simulink model "nextpilot_simulation"  (R2024b)
settings: Solver=FixedStepAuto  StartTime=0.0  StopTime=10.0  FixedStep=5/1000  RelTol=1e-3
libraries: aerolibfltsims x1
settings Model: DataDictionary=nextpilot_datadict.sldd  Creator=zhanfuyu  LastModifiedBy=CETCA
settings SolverCC: MinimalZcImpactIntegration=on
settings OptimizationCC: ReuseModelBlockBuffer=off
settings DebuggingCC: ReadBeforeWriteMsg=DisableAll  WriteAfterWriteMsg=DisableAll  WriteAfterReadMsg=DisableAll  MultiTaskDSMMsg=none
settings ModelReferenceCC: UpdateModelReferenceTargets=IfOutOfDate  EnableParallelModelReferenceBuilds=on
settings SFSimCC: SFSimEcho=off
settings RTWCC: GPUComputeCapability=3.5

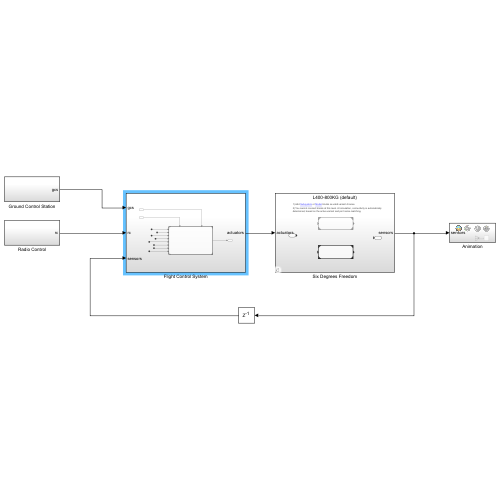
[thumbnail: Simulink's stored preview of the top-level diagram]
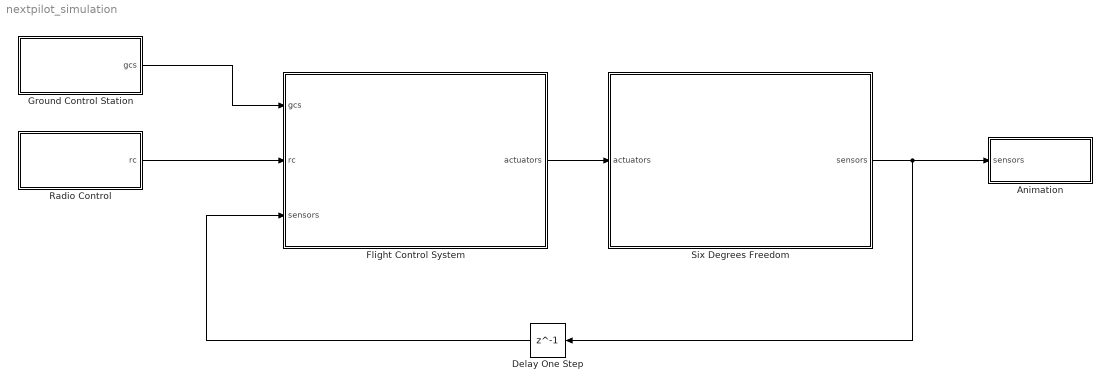
== system nextpilot_simulation ==
  Animation : Subsystem
  Delay One Step : Delay  DelayLength=1
  Flight Control System : Subsystem
  Ground Control Station : Subsystem
  Radio Control : Subsystem
  Six Degrees Freedom : Subsystem  Variant=on
  wires:
  Six Degrees Freedom/1(sensors) -> Delay One Step/1, Animation/1(sensors)
  Radio Control/1(rc) -> Flight Control System/2(rc)
  Ground Control Station/1(gcs) -> Flight Control System/1(gcs)
  Flight Control System/1(actuators) -> Six Degrees Freedom/1(actuators)
  Delay One Step/1 -> Flight Control System/3(sensors)

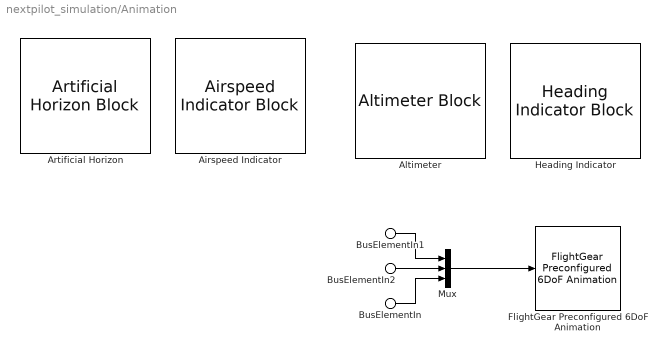
== system nextpilot_simulation/Animation ==
  BusElementIn : Inport  PortName=sensors  Element=states.aircraft.attitude.phi_theta_psi
  BusElementIn1 : Inport  PortName=sensors  Element=states.aircraft.position.lat_lon
  BusElementIn2 : Inport  PortName=sensors  Element=states.aircraft.position.alt
  Airspeed Indicator : AirspeedIndicatorBlock
  Altimeter : AltimeterBlock
  Artificial Horizon : ArtificialHorizonBlock  LabelPosition=Hide
  FlightGear Preconfigured 6DoF Animation : aerolibfltsims/FlightGear Preconfigured 6DoF Animation  xFlightGearVersion=v2019.1  DestinationIpAddress=127.0.0.1  DestinationPort=5502  SampleTime=1/25  packetVersion=24
  Heading Indicator : HeadingIndicatorBlock
  Mux : Mux  Inputs=3
  wires:
  BusElementIn2/1 -> Mux/2
  BusElementIn1/1 -> Mux/1
  BusElementIn/1 -> Mux/3
  Mux/1 -> FlightGear Preconfigured 6DoF Animation/1

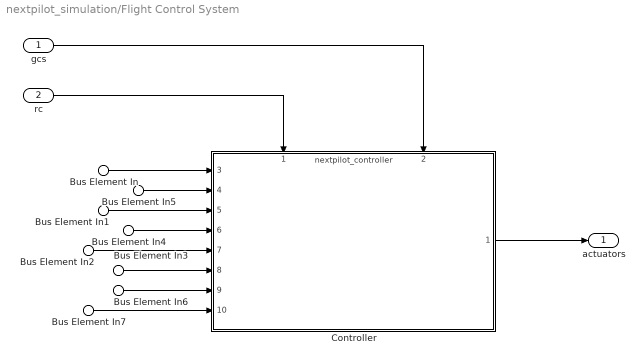
== system nextpilot_simulation/Flight Control System ==
  gcs : Inport
  rc : Inport  Port=2  OutDataTypeStr=Bus: input_rc_s
  Bus Element In : Inport  Port=3  PortName=sensors  Element=gyro
  Bus Element In5 : Inport  Port=3  PortName=sensors  Element=accel
  Bus Element In1 : Inport  Port=3  PortName=sensors  Element=gps
  Bus Element In4 : Inport  Port=3  PortName=sensors  Element=mag
  Bus Element In2 : Inport  Port=3  PortName=sensors  Element=baro
  Bus Element In3 : Inport  Port=3  PortName=sensors  Element=pitot
  Bus Element In6 : Inport  Port=3  PortName=sensors  Element=ahrs
  Bus Element In7 : Inport  Port=3  PortName=sensors  Element=ads
  Controller : ModelReference  ModelNameDialog=nextpilot_controller.slx  SimulationMode=Normal  ModelReferenceVersion=5.48
      settings: PortSchema="{\"entries\":[{\"content\":{\"sides\":[{\"content\":{\"connectorIds\":[\"In3\",\"In4\",\"In5\",\"In6\",\"In7\",\"In8\",\"In9\",\"In10\"]},\"type\":\"ConnectorPlacement.EquallySpacedRectSide\",\"uuid\":\"057d1473-f8ac-40f7-ad61-8fdf511f1a4d\"},{\"content\":{\"connectorIds\":[\"Out1\"],\"side\":\"RIGHT\"},\"type\":\"ConnectorPlacement.EquallySpacedRectSide\",\"uuid\":\"706099eb-7d46-4dab-9c2d-ee6140de84c7\"},{\"content\":{\"connectorIds\":[\"In1\",\"In2\"],\"side\":\"TOP\"},\"type\":\"ConnectorPlacement.EquallySpacedRectSide\",\"uuid\":\"9951fc82-dee5-4b8b-bc13-039f346d1f9b\"}]},\"type\":\"ConnectorPlacement.EquallySpacedConnector\",\"uuid\":\"992bc8bc-323a-4124-b578-9c124df10eb4\"}],\"packageUris\":[\"http://schema.mathworks.com/mf0/Connector/R2020b\"],\"version\":\"1.0\"}"
  actuators : Outport  OutDataTypeStr=Bus: actuator_outputs_s
  wires:
  rc/1 -> Controller/1
  Bus Element In/1 -> Controller/3
  Bus Element In2/1 -> Controller/7
  Bus Element In3/1 -> Controller/8
  Bus Element In4/1 -> Controller/6
  Bus Element In5/1 -> Controller/4
  Bus Element In1/1 -> Controller/5
  gcs/1 -> Controller/2
  Bus Element In6/1 -> Controller/9
  Bus Element In7/1 -> Controller/10
  Controller/1 -> actuators/1

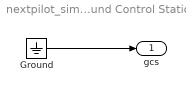
== system nextpilot_simulation/Ground Control Station ==
  Ground : Ground
  gcs : Outport
  wires:
  Ground/1 -> gcs/1

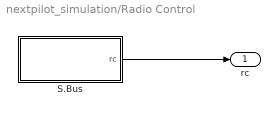
== system nextpilot_simulation/Radio Control ==
  S.Bus : Subsystem
  rc : Outport  OutDataTypeStr=Bus: input_rc_s
  wires:
  S.Bus/1(rc) -> rc/1

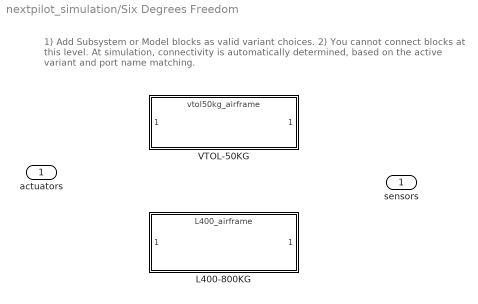
== system nextpilot_simulation/Six Degrees Freedom ==
  note: 1) Add Subsystem or Model blocks as valid variant choices.
      | 2) You cannot connect blocks at this level. At simulation, connectivity is automatically
      | determined, based on the active variant and port name matching.
  actuators : Inport
  L400-800KG : ModelReference  ModelNameDialog=L400_airframe.slx  VariantControl=(default)  ModelReferenceVersion=5.323
  VTOL-50KG : ModelReference  DisableCoverage=on  ModelNameDialog=vtol50kg_airframe.slx  VariantControl=false  ModelReferenceVersion=5.276
  sensors : Outport

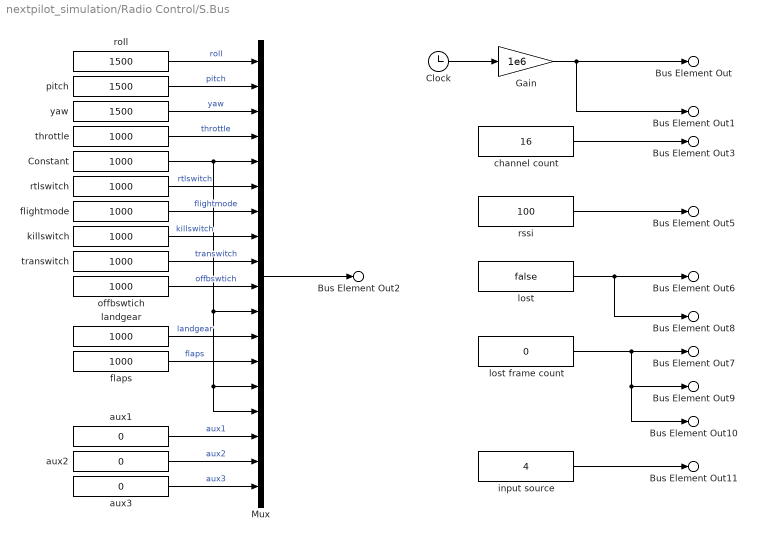
== system nextpilot_simulation/Radio Control/S.Bus ==
  Clock : Clock
  Constant : Constant  Value=1000  OutDataTypeStr=uint16
  Gain : Gain  Gain=1e6  OutDataTypeStr=uint64
  Mux : Mux  Inputs=18
  aux1 : Constant  Value=0  OutDataTypeStr=uint16
  aux2 : Constant  Value=0  OutDataTypeStr=uint16
  aux3 : Constant  Value=0  OutDataTypeStr=uint16
  channel count : Constant  Value=16  OutDataTypeStr=uint8
  flaps : Constant  Value=1000  OutDataTypeStr=uint16
  flightmode : Constant  Value=1000  OutDataTypeStr=uint16
  input source : Constant  Value=4  OutDataTypeStr=uint8
  killswitch : Constant  Value=1000  OutDataTypeStr=uint16
  landgear : Constant  Value=1000  OutDataTypeStr=uint16
  lost : Constant  Value=false  OutDataTypeStr=boolean
  lost frame count : Constant  Value=0  OutDataTypeStr=uint16
  offbswtich : Constant  Value=1000  OutDataTypeStr=uint16
  pitch : Constant  Value=1500  OutDataTypeStr=uint16
  roll : Constant  Value=1500  OutDataTypeStr=uint16
  rssi : Constant  Value=100  OutDataTypeStr=int32
  rtlswitch : Constant  Value=1000  OutDataTypeStr=uint16
  throttle : Constant  Value=1000  OutDataTypeStr=uint16
  transwitch : Constant  Value=1000  OutDataTypeStr=uint16
  yaw : Constant  Value=1500  OutDataTypeStr=uint16
  Bus Element Out : Outport  PortName=rc  Element=timestamp
  Bus Element Out1 : Outport  PortName=rc  Element=timestamp_last_signal
  Bus Element Out3 : Outport  PortName=rc  Element=channel_count
  Bus Element Out5 : Outport  PortName=rc  Element=rssi
  Bus Element Out8 : Outport  PortName=rc  Element=rc_failsafe
  Bus Element Out6 : Outport  PortName=rc  Element=rc_lost
  Bus Element Out7 : Outport  PortName=rc  Element=rc_lost_frame_count
  Bus Element Out9 : Outport  PortName=rc  Element=rc_total_frame_count
  Bus Element Out10 : Outport  PortName=rc  Element=rc_ppm_frame_length
  Bus Element Out11 : Outport  PortName=rc  Element=input_source
  Bus Element Out2 : Outport  PortName=rc  Element=values
  wires:
  Clock/1 -> Gain/1
  Gain/1 -> Bus Element Out1/1, Bus Element Out/1
  channel count/1 -> Bus Element Out3/1
  rssi/1 -> Bus Element Out5/1
  lost frame count/1 -> Bus Element Out10/1, Bus Element Out9/1, Bus Element Out7/1
  lost/1 -> Bus Element Out8/1, Bus Element Out6/1
  input source/1 -> Bus Element Out11/1
  Mux/1 -> Bus Element Out2/1
  roll/1 -> Mux/1  "roll"
  pitch/1 -> Mux/2  "pitch"
  yaw/1 -> Mux/3  "yaw"
  throttle/1 -> Mux/4  "throttle"
  flightmode/1 -> Mux/7  "flightmode"
  killswitch/1 -> Mux/8  "killswitch"
  transwitch/1 -> Mux/9  "transwitch"
  offbswtich/1 -> Mux/10  "offbswtich"
  landgear/1 -> Mux/12  "landgear"
  flaps/1 -> Mux/13  "flaps"
  aux1/1 -> Mux/16  "aux1"
  aux2/1 -> Mux/17  "aux2"
  aux3/1 -> Mux/18  "aux3"
  rtlswitch/1 -> Mux/6  "rtlswitch"
  Constant/1 -> Mux/15, Mux/14, Mux/11, Mux/5
